simulink model "Sim_Ex12"  (R2017a)
settings: Solver=VariableStepAuto  StartTime=0.0  StopTime=Stop_Time  RelTol=1e-3
values from neighbouring files (symbols this model uses):
  I_Ref_Set = [0 10]    [A_Ex12.m]
  Ki = R*Wcc    (= 6283.18530718)    [A_Ex12.m]
  Kp = L*Wcc    (= 6283.18530718)    [A_Ex12.m]
  L = 1    [A_Ex12.m]
  R = 1    [A_Ex12.m]
  Step_Time = 1e-3    (= 0.001)    [A_Ex12.m]
  Wcc = 2*pi*1e3    (= 6283.18530718)    [A_Ex12.m]
settings Model: Creator=KYC  LastModifiedBy=KYC

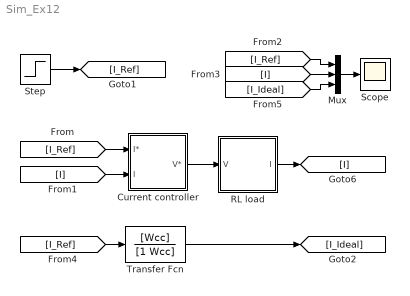
== system Sim_Ex12 ==
  Current controller : Subsystem
  Mux : Mux  Inputs=3
  RL load : Subsystem
  Scope : Scope
  Step : Step  Time=Step_Time  Before=I_Ref_Set(1)  After=I_Ref_Set(2)  SampleTime=0
  Transfer Fcn : TransferFcn  Numerator=[Wcc]  Denominator=[1 Wcc]
  wires:
  Current controller/1(V*) -> RL load/1(V)
  Mux/1 -> Scope/1
  Step/1 -> [I_Ref]
  RL load/1(I) -> [I]
  [I_Ref] -> Current controller/1(I*)
  [I] -> Current controller/2(I)
  [I_Ref] -> Mux/1
  [I] -> Mux/2
  Transfer Fcn/1 -> [I_Ideal]
  [I_Ref] -> Transfer Fcn/1
  [I_Ideal] -> Mux/3

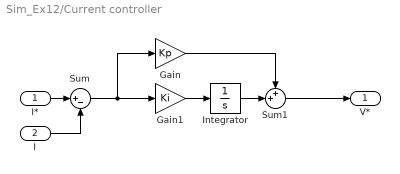
== system Sim_Ex12/Current controller ==
  I* : Inport
  I : Inport  Port=2
  Gain : Gain  Gain=Kp
  Gain1 : Gain  Gain=Ki
  Integrator : Integrator
  Sum : Sum  Inputs=|+-
  Sum1 : Sum  Inputs=++|
  V* : Outport
  wires:
  Gain/1 -> Sum1/1
  Integrator/1 -> Sum1/2
  Gain1/1 -> Integrator/1
  Sum1/1 -> V*/1
  Sum/1 -> Gain/1, Gain1/1
  I*/1 -> Sum/1
  I/1 -> Sum/2

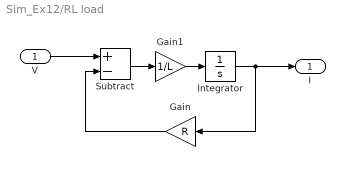
== system Sim_Ex12/RL load ==
  V : Inport
  Gain : Gain  Gain=R
  Gain1 : Gain  Gain=1/L
  Integrator : Integrator
  Subtract : Sum  Inputs=+-
  I : Outport
  wires:
  Subtract/1 -> Gain1/1
  Integrator/1 -> I/1, Gain/1
  Gain/1 -> Subtract/2
  Gain1/1 -> Integrator/1
  V/1 -> Subtract/1
